simulink model "task1"  (R2021a)
settings: Solver=VariableStepAuto  StartTime=0.0  StopTime=10.0  RelTol=1e-3
undefined symbols (not defined in the file or in its folder): Radix
libraries: dspxfrm3 x4
settings Model: Creator=Nadir  LastModifiedBy=Nadir

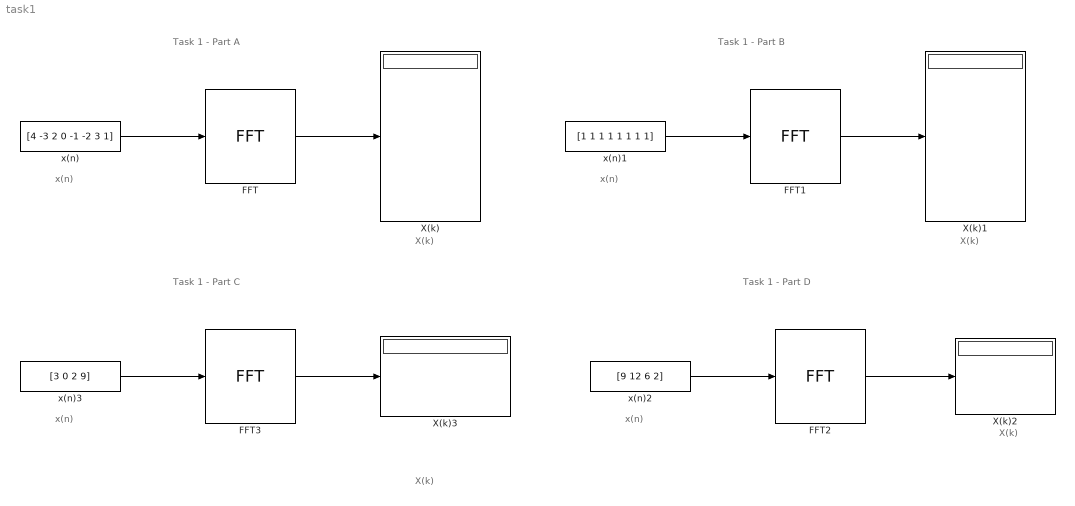
== system task1 ==
  note: x(n)
  note: Task 1 - Part A
  note: X(k)
  note: x(n)
  note: Task 1 - Part B
  note: X(k)
  note: x(n)
  note: Task 1 - Part D
  note: X(k)
  note: x(n)
  note: Task 1 - Part C
  note: X(k)
  FFT{,1..3} (4 alike) : dspxfrm3/FFT  FFTImplementation=Radix-2  CompMethod=Table lookup  TableOpt=NEW  TableOptActive=Speed  BitRevOrder=off  Normalize=off  InheritFFTLength=on  FFTLength=64  WrapInput=on  roundingMode=Floor  overflowMode=off  firstCoeffDataTypeStr=Inherit: Same word length as input  firstCoeffLastDataTypeStr=Inherit: Same word length as input  outputMin=[]  outputMax=[]
  X(k){,1..3} (4 alike) : Display
  x(n) : Constant  Value=[4 -3 2 0 -1 -2 3 1]
  x(n)1 : Constant  Value=[1 1 1 1 1 1 1 1]
  x(n)2 : Constant  Value=[9 12 6 2]
  x(n)3 : Constant  Value=[3 0 2 9]
  wires:
  x(n)/1 -> FFT/1
  FFT/1 -> X(k)/1
  FFT1/1 -> X(k)1/1
  x(n)1/1 -> FFT1/1
  FFT2/1 -> X(k)2/1
  x(n)2/1 -> FFT2/1
  FFT3/1 -> X(k)3/1
  x(n)3/1 -> FFT3/1
